simulink library "INT_Strt_DD"  (R2016b)
settings: Solver=VariableStepAuto  StartTime=0.0  StopTime=10.0  RelTol=1e-3
settings Model: Creator=xuxingpei  LastModifiedBy=xuxingpei

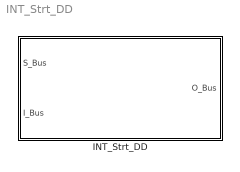
== system INT_Strt_DD ==
  INT_Strt_DD : Subsystem

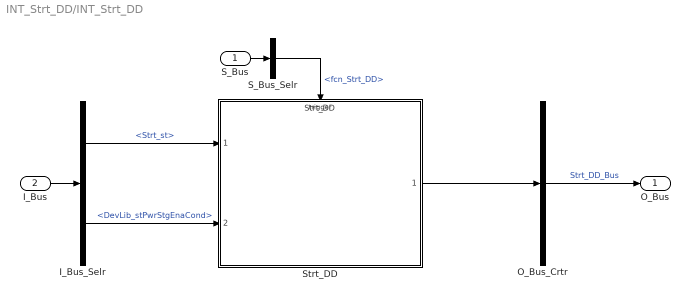
== system INT_Strt_DD/INT_Strt_DD ==
  S_Bus : Inport
  I_Bus : Inport  Port=2
  I_Bus_Selr : BusSelector  OutputSignals=Strt_st,DevLib_stPwrStgEnaCond
  O_Bus_Crtr : BusCreator  Inputs=1
  S_Bus_Selr : BusSelector  OutputSignals=fcn_Strt_DD
  Strt_DD : ModelReference  ModelNameDialog=Strt_DD  SimulationMode=Normal  ModelReferenceVersion=1.15  TriggerPortName=function  TriggerPortTriggerType=function-call  TriggerPortStatesWhenEnabling=held
  O_Bus : Outport
  wires:
  S_Bus_Selr/1 -> Strt_DD/Trigger  "<fcn_Strt_DD>"
  S_Bus/1 -> S_Bus_Selr/1
  I_Bus/1 -> I_Bus_Selr/1
  I_Bus_Selr/1 -> Strt_DD/1  "<Strt_st>"
  I_Bus_Selr/2 -> Strt_DD/2  "<DevLib_stPwrStgEnaCond>"
  O_Bus_Crtr/1 -> O_Bus/1  "Strt_DD_Bus"
  Strt_DD/1 -> O_Bus_Crtr/1
